simulink subsystem "ServoSimulation"  (R2019b)
settings: Solver=VariableStepAuto  StartTime=0.0  StopTime=10.0  RelTol=1e-3
libraries: simulink x2
settings Model: Creator=toons  LastModifiedBy=toons

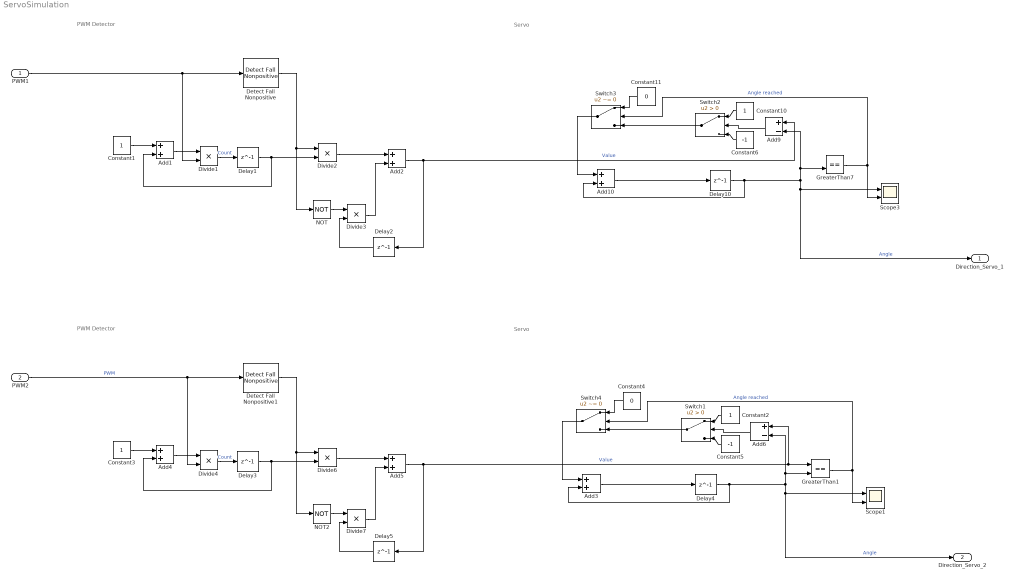
== system ServoSimulation ==
  note: PWM Detector
  note: Servo
  note: Servo
  note: PWM Detector
  PWM1 : Inport
  PWM2 : Inport  Port=2
  Add{1..5,10} (6 alike) : Sum
  Add6 : Sum  Inputs=+-
  Add9 : Sum  Inputs=+-
  Constant{1..3,10} (4 alike) : Constant
  Constant11 : Constant  Value=0
  Constant4 : Constant  Value=0
  Constant5 : Constant  Value=-1
  Constant6 : Constant  Value=-1
  Delay{1..3,5} (4 alike) : Delay  DelayLength=1  SampleTime=1/12800
  Delay10 : Delay  DelayLength=1  SampleTime=0.16/60
  Delay4 : Delay  DelayLength=1  SampleTime=0.16/60
  Detect Fall Nonpositive : simulink/Logic and Bit Operations/Detect Fall Nonpositive  vinit=1  OutDataTypeStr=boolean
      settings: SourceProductName=Simulink  SourceProductBaseCode=SL
  Detect Fall Nonpositive1 : simulink/Logic and Bit Operations/Detect Fall Nonpositive  vinit=1  OutDataTypeStr=boolean
      settings: SourceProductName=Simulink  SourceProductBaseCode=SL
  Divide1 : Product  Inputs=**  SaturateOnIntegerOverflow=on  RndMeth=Zero
  Divide{2..3,6..7} (4 alike) : Product  Inputs=**
  Divide4 : Product  Inputs=**  SaturateOnIntegerOverflow=on  RndMeth=Zero
  GreaterThan1 : RelationalOperator  Operator===  OutDataTypeStr=boolean  RndMeth=Simplest
  GreaterThan7 : RelationalOperator  Operator===  OutDataTypeStr=boolean  RndMeth=Simplest
  NOT : Logic  Operator=NOT  IconShape=distinctive  AllPortsSameDT=off  OutDataTypeStr=boolean
  NOT2 : Logic  Operator=NOT  IconShape=distinctive  AllPortsSameDT=off  OutDataTypeStr=boolean
  Scope1 : Scope  NumInputPorts=2
  Scope3 : Scope  NumInputPorts=2
  Switch1 : Switch  Criteria=u2 > Threshold
  Switch2 : Switch  Criteria=u2 > Threshold
  Switch3 : Switch  Criteria=u2 ~= 0
  Switch4 : Switch  Criteria=u2 ~= 0
  Direction_Servo_1 : Outport
  Direction_Servo_2 : Outport  Port=2
  wires:
  Divide3/1 -> Add2/2
  NOT/1 -> Divide3/1
  Divide2/1 -> Add2/1
  Delay1/1 -> Divide2/2, Add1/2
  Delay3/1 -> Divide6/2, Add4/2
  Detect Fall Nonpositive/1 -> NOT/1, Divide2/1
  Divide6/1 -> Add5/1
  Constant3/1 -> Add4/1
  Divide4/1 -> Delay3/1  "Count"
  Delay5/1 -> Divide7/2
  NOT2/1 -> Divide7/1
  Divide7/1 -> Add5/2
  Divide1/1 -> Delay1/1  "Count"
  PWM1/1 -> Divide1/2, Detect Fall Nonpositive/1
  Add1/1 -> Divide1/1
  Delay2/1 -> Divide3/2
  PWM2/1 -> Detect Fall Nonpositive1/1, Divide4/2  "PWM"
  Constant1/1 -> Add1/1
  Add4/1 -> Divide4/1
  Detect Fall Nonpositive1/1 -> NOT2/1, Divide6/1
  Constant6/1 -> Switch2/3
  Switch3/1 -> Add10/1
  Constant11/1 -> Switch3/1
  Add9/1 -> Switch2/2
  Add10/1 -> Delay10/1
  Switch2/1 -> Switch3/3
  GreaterThan7/1 -> Switch3/2, Scope3/2  "Angle reached"
  Delay10/1 -> Scope3/1, Direction_Servo_1/1, GreaterThan7/2, Add9/2, Add10/2  "Angle"
  Add2/1 -> Delay2/1, Add9/1  "Value"
  Constant10/1 -> Switch2/1
  Delay4/1 -> Scope1/1, Direction_Servo_2/1, GreaterThan1/2, Add6/2, Add3/2  "Angle"
  Add5/1 -> GreaterThan1/1, Add6/1, Delay5/1  "Value"
  Constant2/1 -> Switch1/1
  Switch4/1 -> Add3/1
  Add3/1 -> Delay4/1
  Constant4/1 -> Switch4/1
  Add6/1 -> Switch1/2
  Constant5/1 -> Switch1/3
  GreaterThan1/1 -> Switch4/2, Scope1/2  "Angle reached"
  Switch1/1 -> Switch4/3
